simulink model "MotorXploer"  (R2024b)
settings: Solver=FixedStepAuto  StartTime=0.0  StopTime=inf  FixedStep=0.0001  RelTol=1e-3  EnableMultiTasking=on
undefined symbols (not defined in the file): Blocking, LF, Non
libraries: hdlsllib x5, simulink x4, amg_usbconverter_n_connect_lib x3
settings Model: Creator=beamk  LastModifiedBy=A1nz_01
settings OptimizationCC: DefaultParameterBehavior=Inlined  EnhancedBackFolding=on  PassReuseOutputArgsAs=Individual arguments  ZeroExternalMemoryAtStartup=off  ZeroInternalMemoryAtStartup=off  MaxStackSize=512  OptimizeBlockOrder=speed  DifferentSizesBufferReuse=on  OptimizationCustomize=off  EfficientTunableParamExpr=on
settings DebuggingCC: ParameterTunabilityLossMsg=error
settings SFSimCC: MATLABDynamicMemAlloc=off
settings RTWCC: Description=Embedded Coder  SystemTargetFile=ert.tlc  TemplateMakefile=ert_default_tmf  Toolchain=GNU Tools for ARM Embedded Processors
settings CodeAppCC: ForceParamTrailComments=on  IgnoreCustomStorageClasses=off  OperatorAnnotations=on  SimulinkDataObjDesc=on  SFDataObjDesc=on  InsertBlockDesc=on
settings ERTTargetCC: TargetLangStandard=C99 (ISO)  CodeReplacementLibrary=ARM Cortex-M  ExtModeTransport=3  ExtModeStaticAlloc=on  ExtModeStaticAllocSize=2048  ExtModeMexFile=ext_xcp  ExtModeIntrfLevel=Level2 - Open  ERTCustomFileTemplate=example_file_process.tlc

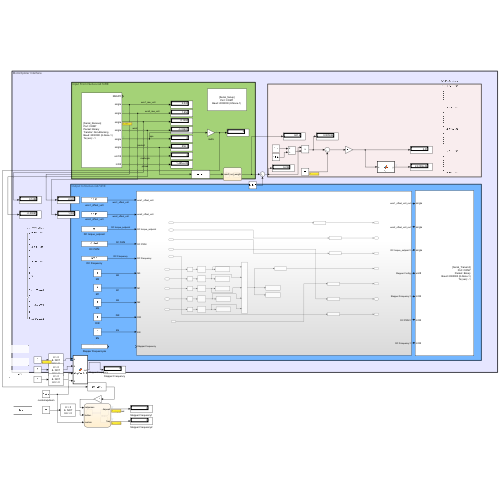
[thumbnail: Simulink's stored preview of the top-level diagram]
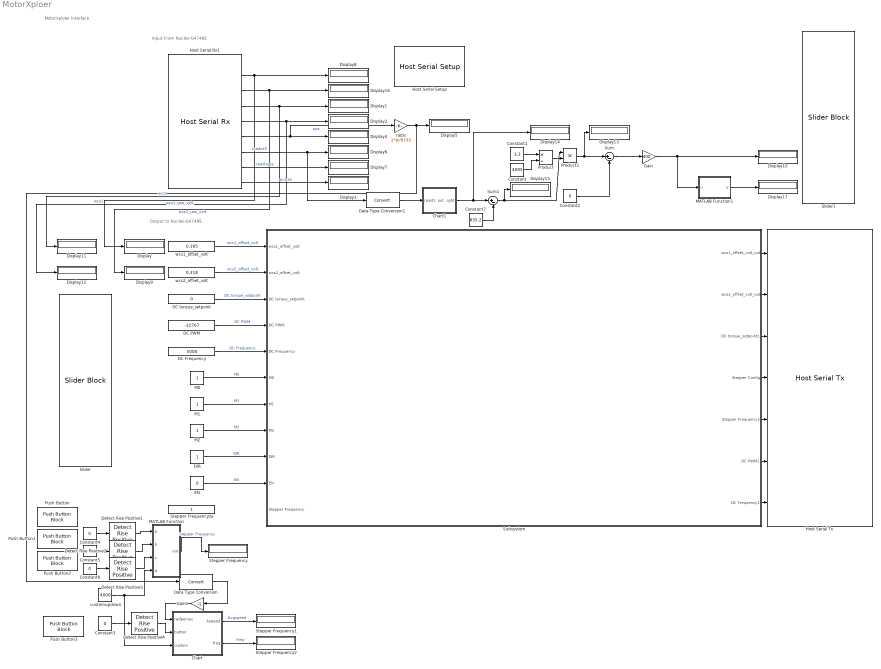
== system MotorXploer ==
  note: Output to Nucleo-G474RE
  note: Input From Nucleo-G474RE
  note: MotorXploler Interface
  Chart : Stateflow chart  TreatAsAtomicUnit=on
      settings: PortSchema="{\"entries\":[{\"content\":{\"sides\":[{\"content\":{\"connectorIds\":[\"In3\",\"In1\",\"In2\"]},\"type\":\"ConnectorPlacement.EquallySpacedRectSide\",\"uuid\":\"0af0ecde-5d05-4581-bcd2-08afd14d6a73\"},{\"content\":{\"connectorIds\":[\"Out1\",\"Out2\"],\"side\":\"RIGHT\"},\"type\":\"ConnectorPlacement.EquallySpacedRectSide\",\"uuid\":\"b178b433-65d2-4053-becb-82ca8e4817f3\"},{\"content\":{\"side\":\"TOP\"},\"type\":\"ConnectorPlacement.EquallySpacedRectSide\",\"uuid\":\"5242ac66-5f55-46dd-8c60-bf54cb5bba4a\"}]},\"type\":\"ConnectorPlacement.EquallySpacedConnector\",\"uuid\":\"06805e83-7497-4c5c-8fd4-48f89936d5b4\"}],\"packageUris\":[\"http://schema.mathworks.com/mf0/Connector/R2020b\"],\"version\":\"1.0\"}"
  Chart1 : Stateflow chart  TreatAsAtomicUnit=on
  Constant : Constant  Value=4095
  Constant1 : Constant  Value=3.3
  Constant{2..6} (5 alike) : Constant  Value=0
  Constant7 : Constant  Value=835.2
  DC Frequency : Constant  Value=5000
  DC PWM : Constant  Value=-32767
  DC torque_setpoint : Constant  Value=0
  DIR : Constant  OutDataTypeStr=uint8
  Data Type Conversion : DataTypeConversion  SaturateOnIntegerOverflow=off  RndMeth=Floor
  Data Type Conversion1 : DataTypeConversion  SaturateOnIntegerOverflow=off  RndMeth=Floor
  Detect Rise Positive{1..4} (4 alike) : simulink/Logic and Bit Operations/Detect Rise Positive  vinit=0  OutDataTypeStr=boolean
  Display{,1..17} (18 alike) : Display
      Display17 settings: Format=short_e
  EN : Constant  Value=0  OutDataTypeStr=uint8
  Gain : Gain  Gain=400
  Gain1 : Gain  Gain=-1
  Host Serial Rx1 : amg_usbconverter_n_connect_lib/Host Serial Rx  conf=rx  port=COM7  baudrate=2000000  databits=8  parity=None  stopbit=1  flowcontrol=None  transfer=Non-Blocking  timeout=5  packetmode=Binary  enableinitialvalues=off  initialvalues=[]  binheader='45'  binterminator='A'  porttype_double=0  porttype_single=6  porttype_int8=0  porttype_uint8=0  porttype_int16=0  porttype_uint16=1  porttype_int32=1  porttype_uint32=0  asciiformat='%f,%f,%d,%d'  rx_asciiterminator="LF (0x0A - \"\\n\")"  tx_asciiterminator="CRLF (0x0D 0x0A - \"\\r\\n\")"  sampletime=-1  enablecustomportlabel=off  cinputportlabel=0  coutputportlabel=A  portpinstr=0  blockid=HostSerialRx1  inputporttype=[]  inputportwidth=[]  inputportlabel={}  outputporttype=[3 1 1 1 1 1 1 5 6]  outputportwidth=[1 1 1 1 1 1 1 1 1]  outputportlabel={'READY','single','single','single','single','single','single','uint16','int32'}  compat=0  optionstring=[]  autoport='COM7'
  Host Serial Setup : amg_usbconverter_n_connect_lib/Host Serial Setup  conf=setup  port=COM7  baudrate=2000000  databits=8  parity=None  stopbit=1  flowcontrol=None  transfer=Blocking  timeout=2  packetmode=Binary  initialvalues=[]  binheader='7E 7E'  binterminator='03 03'  porttype_double=0  porttype_single=1  porttype_int8=0  porttype_uint8=0  porttype_int16=0  porttype_uint16=0  porttype_int32=0  porttype_uint32=2  asciiformat='%d %u %x'  rx_asciiterminator="CRLF (0x0D 0x0A - \"\\r\\n\")"  tx_asciiterminator="CRLF (0x0D 0x0A - \"\\r\\n\")"  sampletime=-1  enablecustomportlabel=off  cinputportlabel=0  coutputportlabel=A  portpinstr=0  blockid=HostSerialSetup  inputporttype=[]  inputportwidth=[]  inputportlabel={}  outputporttype=[]  outputportwidth=[]  outputportlabel={}  compat=0  optionstring=[]  autoport='COM7'
  Host Serial Tx : amg_usbconverter_n_connect_lib/Host Serial Tx  conf=tx  port=COM7  baudrate=2000000  databits=8  parity=None  stopbit=1  flowcontrol=None  transfer=Blocking  timeout=2  packetmode=Binary  initialvalues=[]  binheader='45'  binterminator='A'  porttype_double=0  porttype_single=3  porttype_int8=0  porttype_uint8=1  porttype_int16=0  porttype_uint16=0  porttype_int32=3  porttype_uint32=0  asciiformat='%d,%f'  rx_asciiterminator="CRLF (0x0D 0x0A - \"\\r\\n\")"  tx_asciiterminator="CRLF (0x0D 0x0A - \"\\r\\n\")"  sampletime=-1  enablecustomportlabel=off  cinputportlabel=0  coutputportlabel=A  portpinstr=0  blockid=HostSerialTx  inputporttype=[1 1 1 3 6 6 6]  inputportwidth=[1 1 1 1 1 1 1]  inputportlabel={'single','single','single','uint8','int32','int32','int32'}  outputporttype=[]  outputportwidth=[]  outputportlabel={}  compat=0  optionstring=[]  autoport='COM7'
      settings: SourceProductName=aMG USB Converter N
  M0 : Constant  OutDataTypeStr=uint8
  M1 : Constant  OutDataTypeStr=uint8
  M2 : Constant  OutDataTypeStr=uint8
  MATLAB Function : MATLAB Function  TreatAsAtomicUnit=on
  MATLAB Function1 : MATLAB Function  TreatAsAtomicUnit=on
  Product : Product  Inputs=*/
  Product1 : Product
  Push Button : PushButtonBlock  ButtonText=+  OffValue=0.000000
  Push Button1 : PushButtonBlock  ButtonText=-  OffValue=0.000000
  Push Button2 : PushButtonBlock  ButtonText=1000  OffValue=0.000000
  Push Button3 : PushButtonBlock  OffValue=0.000000
  Slider : SliderBlock  ScaleMin=-65535  ScaleMax=65535
  Slider1 : SliderBlock  ScaleMin=-65535  ScaleMax=-32767
  Stepper Frequency : Display
  Stepper Frequency1 : Display
  Stepper Frequency2 : Display
  Stepper Frequencyza : Constant
  Subsystem : Subsystem
  Sum : Sum  Inputs=|+-
  Sum1 : Sum  Inputs=|+-
  customupdown : Constant  Value=4000
  rad/s : Gain  Gain=2*pi/8192
  wcs1_offset_volt : Constant  Value=0.395  OutDataTypeStr=single
  wcs2_offset_volt : Constant  Value=0.318  OutDataTypeStr=single
  wires:
  Host Serial Rx1/2 -> Display/1, Display8/1  "wcs1_raw_volt"
  Host Serial Rx1/3 -> Display9/1, Display16/1  "wcs2_raw_volt"
  Host Serial Rx1/7 -> Data Type Conversion1/1, Display6/1  "loadcell"
  Host Serial Rx1/5 -> Display12/1, Display2/1  "wcs2"
  Host Serial Rx1/8 -> Display7/1  "rawAngle"
  rad/s/1 -> Data Type Conversion/1, Display5/1
  Host Serial Rx1/6 -> Display4/1, rad/s/1  "pps"
  Host Serial Rx1/9 -> Display3/1  "pulses"
  wcs1_offset_volt/1 -> Subsystem/1(wcs1_offset_volt)  "wcs1_offset_volt"
  wcs2_offset_volt/1 -> Subsystem/2(wcs2_offset_volt)  "wcs2_offset_volt"
  DC torque_setpoint/1 -> Subsystem/3(DC torque_setpoint)  "DC torque_setpoint"
  DC PWM/1 -> Subsystem/4(DC PWM)  "DC PWM"
  DC Frequency/1 -> Subsystem/5(DC Frequency)  "DC Frequency"
  M0/1 -> Subsystem/6(M0)  "M0"
  M1/1 -> Subsystem/7(M1)  "M1"
  M2/1 -> Subsystem/8(M2)  "M2"
  DIR/1 -> Subsystem/9(DIR)  "DIR"
  EN/1 -> Subsystem/10(EN)  "EN"
  Subsystem/1(wcs1_offset_volt_out) -> Host Serial Tx/1
  Subsystem/2(wcs2_offset_volt_out) -> Host Serial Tx/2
  Subsystem/3(DC torque_setpoint1) -> Host Serial Tx/3
  Subsystem/4(Stepper Config) -> Host Serial Tx/4
  Subsystem/5(Stepper Frequency1) -> Host Serial Tx/5
  Subsystem/6(DC PWM1) -> Host Serial Tx/6
  Subsystem/7(DC Frequency1) -> Host Serial Tx/7
  Product/1 -> Product1/2
  Constant/1 -> Product/2
  Constant1/1 -> Product/1
  Constant2/1 -> Sum/2
  Product1/1 -> Display13/1, Sum/1
  Sum/1 -> Gain/1
  Constant4/1 -> Detect Rise Positive1/1
  MATLAB Function/1(out) -> Stepper Frequency/1  "Stepper Frequency"
  Constant6/1 -> Detect Rise Positive3/1
  Constant5/1 -> Detect Rise Positive2/1
  Detect Rise Positive1/1 -> MATLAB Function/1(a)
  Detect Rise Positive2/1 -> MATLAB Function/2(b)
  Detect Rise Positive3/1 -> MATLAB Function/3(c)
  customupdown/1 -> Chart/2(custom), MATLAB Function/4(d)
  Constant3/1 -> Detect Rise Positive4/1
  Detect Rise Positive4/1 -> Chart/1(button)
  Chart/1(Aspeed) -> Stepper Frequency1/1  "Avgspeed"
  Chart/2(freq) -> Stepper Frequency2/1  "freq"
  Data Type Conversion/1 -> Gain1/1
  Gain1/1 -> Chart/3(radpersec)
  Host Serial Rx1/4 -> Display11/1, Display1/1  "wcs1"
  Constant7/1 -> Sum1/2
  Sum1/1 -> Display15/1, Product1/1
  MATLAB Function1/1(y) -> Display17/1
  Chart1/1(out_weight) -> Display14/1, Sum1/1
  Gain/1 -> Display10/1, MATLAB Function1/1(u)
  Data Type Conversion1/1 -> Chart1/1(read1)

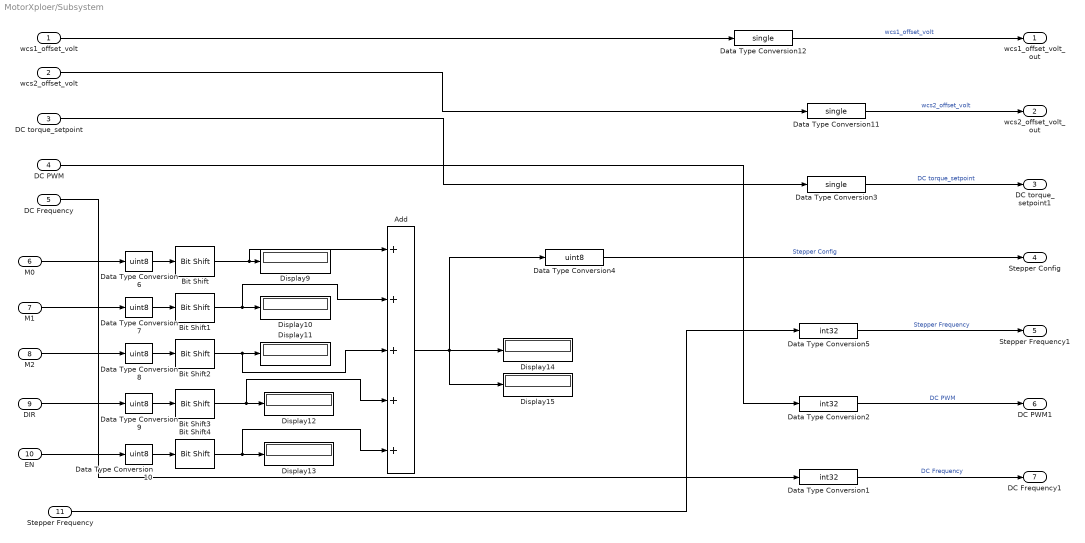
== system MotorXploer/Subsystem ==
  wcs1_offset_volt : Inport
  wcs2_offset_volt : Inport  Port=2
  DC torque_setpoint : Inport  Port=3
  DC PWM : Inport  Port=4
  DC Frequency : Inport  Port=5
  M0 : Inport  Port=6
  M1 : Inport  Port=7
  M2 : Inport  Port=8
  DIR : Inport  Port=9
  EN : Inport  Port=10
  Stepper Frequency : Inport  Port=11
  Add : Sum  Inputs=+++++
  Bit Shift : hdlsllib/Logic and Bit Operations/Bit Shift  mode=Shift Left Logical  N=4
  Bit Shift1 : hdlsllib/Logic and Bit Operations/Bit Shift  mode=Shift Left Logical  N=3
  Bit Shift2 : hdlsllib/Logic and Bit Operations/Bit Shift  mode=Shift Left Logical  N=2
  Bit Shift3 : hdlsllib/Logic and Bit Operations/Bit Shift  mode=Shift Left Logical  N=1
  Bit Shift4 : hdlsllib/Logic and Bit Operations/Bit Shift  mode=Shift Left Logical  N=0
  Data Type Conversion1 : DataTypeConversion  OutDataTypeStr=int32  SaturateOnIntegerOverflow=off  RndMeth=Floor
  Data Type Conversion{4,6..10} (6 alike) : DataTypeConversion  OutDataTypeStr=uint8  SaturateOnIntegerOverflow=off  RndMeth=Floor
  Data Type Conversion11 : DataTypeConversion  OutDataTypeStr=single  SaturateOnIntegerOverflow=off  RndMeth=Floor
  Data Type Conversion12 : DataTypeConversion  OutDataTypeStr=single  SaturateOnIntegerOverflow=off  RndMeth=Floor
  Data Type Conversion2 : DataTypeConversion  OutDataTypeStr=int32  SaturateOnIntegerOverflow=off  RndMeth=Floor
  Data Type Conversion3 : DataTypeConversion  OutDataTypeStr=single  SaturateOnIntegerOverflow=off  RndMeth=Floor
  Data Type Conversion5 : DataTypeConversion  OutDataTypeStr=int32  SaturateOnIntegerOverflow=off  RndMeth=Floor
  Display{9..15} (7 alike) : Display
      Display10 settings: Format=binary (Stored Integer)
      Display11 settings: Format=binary (Stored Integer)
      Display12 settings: Format=binary (Stored Integer)
      Display13 settings: Format=binary (Stored Integer)
      Display14 settings: Format=binary (Stored Integer)
      Display9 settings: Format=binary (Stored Integer)
  wcs1_offset_volt_out : Outport
  wcs2_offset_volt_out : Outport  Port=2
  DC torque_setpoint1 : Outport  Port=3
  Stepper Config : Outport  Port=4
  Stepper Frequency1 : Outport  Port=5
  DC PWM1 : Outport  Port=6
  DC Frequency1 : Outport  Port=7
  wires:
  Bit Shift/1 -> Display9/1, Add/1
  Data Type Conversion8/1 -> Bit Shift2/1
  EN/1 -> Data Type Conversion10/1
  Data Type Conversion6/1 -> Bit Shift/1
  DC torque_setpoint/1 -> Data Type Conversion3/1
  Data Type Conversion2/1 -> DC PWM1/1  "DC PWM"
  Data Type Conversion7/1 -> Bit Shift1/1
  Data Type Conversion10/1 -> Bit Shift4/1
  DC PWM/1 -> Data Type Conversion2/1
  Bit Shift3/1 -> Display12/1, Add/4
  Data Type Conversion12/1 -> wcs1_offset_volt_out/1  "wcs1_offset_volt"
  Add/1 -> Display15/1, Display14/1, Data Type Conversion4/1
  Bit Shift2/1 -> Display11/1, Add/3
  Stepper Frequency/1 -> Data Type Conversion5/1
  M1/1 -> Data Type Conversion7/1
  Bit Shift1/1 -> Display10/1, Add/2
  Bit Shift4/1 -> Display13/1, Add/5
  M0/1 -> Data Type Conversion6/1
  Data Type Conversion9/1 -> Bit Shift3/1
  Data Type Conversion11/1 -> wcs2_offset_volt_out/1  "wcs2_offset_volt"
  M2/1 -> Data Type Conversion8/1
  wcs1_offset_volt/1 -> Data Type Conversion12/1
  DC Frequency/1 -> Data Type Conversion1/1
  wcs2_offset_volt/1 -> Data Type Conversion11/1
  Data Type Conversion1/1 -> DC Frequency1/1  "DC Frequency"
  DIR/1 -> Data Type Conversion9/1
  Data Type Conversion4/1 -> Stepper Config/1  "Stepper Config"
  Data Type Conversion3/1 -> DC torque_setpoint1/1  "DC torque_setpoint"
  Data Type Conversion5/1 -> Stepper Frequency1/1  "Stepper Frequency"

== matlab function MotorXploer/MATLAB Function1 ==
  data: u input; y output
function y = fcn(u)
b = u*(0.01);
a = deg2rad(6.76);
y = b*sin(a)*0.1105;

== matlab function MotorXploer/MATLAB Function ==
  data: a input; out output; b input; c input; d input
function out = stepControl(a,b,c,d)
if(a == 1)
    action = -1;
elseif(b == 1)
    action = -2;
elseif(c == 1)
    action = -3;
else
    action = 0;
end
% action: ค่าจากปุ่ม (-1, 0, 1)
% currentValue: ค่าปัจจุบัน
% out: ค่าที่อัปเดต
check = 0;
persistent value; % ค่าที่เก็บสถานะ
if isempty(value)
    value = 0; % ค่าเริ่มต้น
end

switch action
    case -1 % ปุ่ม +100
        if(check==0)
            check=1;
            value = value + d;
        end
    case -2 % ปุ่ม -100
        if(check==0)
            check=1;
            value = value - d;
        end
    case -3 % ปุ่ม Reset
        if(check==0)
            check=1;
            value = 1000;
        end
end
if(action~=-1&&action~=2&&action~=3)
    check = 0;
end


out = value;
end

== stateflow chart MotorXploer/Chart ==
  state Init
    freq = 0;
    time = 0;
    oldspeed = 0;
    Aspeed = 0;
    timecount = 0;
    oldspeed = radpersec;
    checkpoint =0;
    exit:
    time = 0;
  state start
    during:
    time = time+0.0001;
    timecount = timecount+0.0001;
    checkpoint = checkpoint+radpersec;
    exit:
    Aspeed = checkpoint/10000
  state upscale
    exit:
    freq = freq+custom;
    timecount =0;
  (default) -> Init
  Init -> start : [button ==1]
  start -> Init [order 2] : [radpersec < 1 && time>2]
  upscale -> start
  start -> upscale [order 1] : [timecount >  1]
  data: button input; custom input; radpersec input; Aspeed output; freq output; time local; oldspeed local; timecount local; checkpoint local

== stateflow chart MotorXploer/Chart1 ==
  state init
    time = 0;
    weight = 0;
    read = read1;
    entry:
    time = 0;
  state avg
    entry:
    weight = 0;
    during:
    weight = weight+read;
    time = time+0.0001;
    exit:
    out_weight = weight/10000;
  (default) -> init
  init -> avg
  avg -> init : [time > 1]
  data: out_weight output; time local; weight local; read local; read1 input
